simulink model "Linearisation_AleixGranero_MichalSzabo"  (R2021b)
settings: Solver=ode3  StartTime=0.0  StopTime=1000  FixedStep=Ts  RelTol=1e-3  EnableMultiTasking=on
values from neighbouring files (symbols this model uses):
  A = [K1   0 -K3   0 ... (first row only)    [Discretisation_MichalSzabo_AleixGranero.m]    (also in Linearisation_MichalSzabo_AleixGranero.m)
  A1 = 28    [Discretisation_MichalSzabo_AleixGranero.m]    (also in Linearisation_MichalSzabo_AleixGranero.m)
  a1 = 0.071    [Discretisation_MichalSzabo_AleixGranero.m]    (also in Linearisation_MichalSzabo_AleixGranero.m)
  A2 = 28    [Discretisation_MichalSzabo_AleixGranero.m]    (also in Linearisation_MichalSzabo_AleixGranero.m)
  a2 = 0.071    [Discretisation_MichalSzabo_AleixGranero.m]    (also in Linearisation_MichalSzabo_AleixGranero.m)
  a3 = 0.071    [Discretisation_MichalSzabo_AleixGranero.m]    (also in Linearisation_MichalSzabo_AleixGranero.m)
  A3 = 28    [Discretisation_MichalSzabo_AleixGranero.m]    (also in Linearisation_MichalSzabo_AleixGranero.m)
  a4 = 0.071    [Discretisation_MichalSzabo_AleixGranero.m]    (also in Linearisation_MichalSzabo_AleixGranero.m)
  A4 = 28    [Discretisation_MichalSzabo_AleixGranero.m]    (also in Linearisation_MichalSzabo_AleixGranero.m)
  B = [J2 0 ... (first row only)    [Discretisation_MichalSzabo_AleixGranero.m]    (also in Linearisation_MichalSzabo_AleixGranero.m)
  C = eye(4)    [Discretisation_MichalSzabo_AleixGranero.m]    (also in Linearisation_MichalSzabo_AleixGranero.m)
  D = zeros(4,2)    [Discretisation_MichalSzabo_AleixGranero.m]    (also in Linearisation_MichalSzabo_AleixGranero.m)
  g = 981    [Discretisation_MichalSzabo_AleixGranero.m]    (also in Linearisation_MichalSzabo_AleixGranero.m)
  gamma1 = 0.7    [Discretisation_MichalSzabo_AleixGranero.m]    (also in Linearisation_MichalSzabo_AleixGranero.m)
  gamma2 = 0.7    [Discretisation_MichalSzabo_AleixGranero.m]    (also in Linearisation_MichalSzabo_AleixGranero.m)
  h10 = 1/(2*g)*(a3/a1 * sqrt(2*g*h30)+gamma1*k1/a1*v10)^2    [Discretisation_MichalSzabo_AleixGranero.m]    (also in Linearisation_MichalSzabo_AleixGranero.m)
  h20 = 1/(2*g)*(a4/a2 * sqrt(2*g*h40)+gamma2*k1/a2*v20)^2    [Discretisation_MichalSzabo_AleixGranero.m]    (also in Linearisation_MichalSzabo_AleixGranero.m)
  h30 = 1/(2*g)*((1-gamma2)*k2*v20/a3)^2    (= 0.40362240636)    [Discretisation_MichalSzabo_AleixGranero.m]    (also in Linearisation_MichalSzabo_AleixGranero.m)
  h40 = 1/(2*g)*((1-gamma1)*k2*v10/a4)^2    (= 0.40362240636)    [Discretisation_MichalSzabo_AleixGranero.m]    (also in Linearisation_MichalSzabo_AleixGranero.m)
  k1 = 3.33    [Discretisation_MichalSzabo_AleixGranero.m]    (also in Linearisation_MichalSzabo_AleixGranero.m)
  k2 = 3.33    [Discretisation_MichalSzabo_AleixGranero.m]    (also in Linearisation_MichalSzabo_AleixGranero.m)
  t1 = 200    [Discretisation_MichalSzabo_AleixGranero.m]    (also in Linearisation_MichalSzabo_AleixGranero.m)
  t2 = 400    [Discretisation_MichalSzabo_AleixGranero.m]    (also in Linearisation_MichalSzabo_AleixGranero.m)
  v10 = 2    [Discretisation_MichalSzabo_AleixGranero.m]    (also in Linearisation_MichalSzabo_AleixGranero.m)
  v11 = 2.2    [Discretisation_MichalSzabo_AleixGranero.m]    (also in Linearisation_MichalSzabo_AleixGranero.m)
  v20 = 2    [Discretisation_MichalSzabo_AleixGranero.m]    (also in Linearisation_MichalSzabo_AleixGranero.m)
  v22 = 1.8    [Discretisation_MichalSzabo_AleixGranero.m]    (also in Linearisation_MichalSzabo_AleixGranero.m)
settings Model: Creator=as  LastModifiedBy=szmis
settings SolverCC: AlgebraicLoopSolver=TrustRegion
settings DataIOCC: LimitDataPoints=on  SaveFormat=Array  SignalLoggingSaveFormat=ModelDataLogs  ReturnWorkspaceOutputs=off
settings OptimizationCC: LifeSpan=inf
settings DebuggingCC: SaveWithParameterizedLinksMsg=none  UnderspecifiedInitializationDetection=Classic  MergeDetectMultiDrivingBlocksExec=none  SolverPrmCheckMsg=warning  FcnCallInpInsideContextMsg=warning  SFUnexpectedBacktrackingDiag=warning  SFNoUnconditionalDefaultTransitionDiag=warning  SFExecutionAtInitializationDiag=none  SFMachineParentedDataDiag=warning  ArithmeticOperatorsInVariantConditions=warning
settings HardwareCC: ProdBitPerPointer=32  ProdBitPerSizeT=32  ProdBitPerPtrDiffT=32  ProdLargestAtomicFloat=None  ProdIntDivRoundTo=Undefined  ProdEndianess=Unspecified  ProdWordSize=32  ProdHWDeviceType=32-bit Generic
settings ModelReferenceCC: PropagateSignalLabelsOutOfModel=off
settings SFSimCC: SimUseLocalCustomCode=off  CustomCodeUndefinedFunction=UseInterfaceOnly
settings RTWCC: RTWUseLocalCustomCode=off
settings CodeAppCC: StateflowObjectComments=on
settings GRTTargetCC: TargetLangStandard=C89/C90 (ANSI)  CombineOutputUpdateFcns=off  GRTInterface=on
settings ConfigComp: CovMetricSettings=dw  CovSaveCumulativeToWorkspaceVar=on  CovSaveSingleToWorkspaceVar=on  CovExternalEMLEnable=off

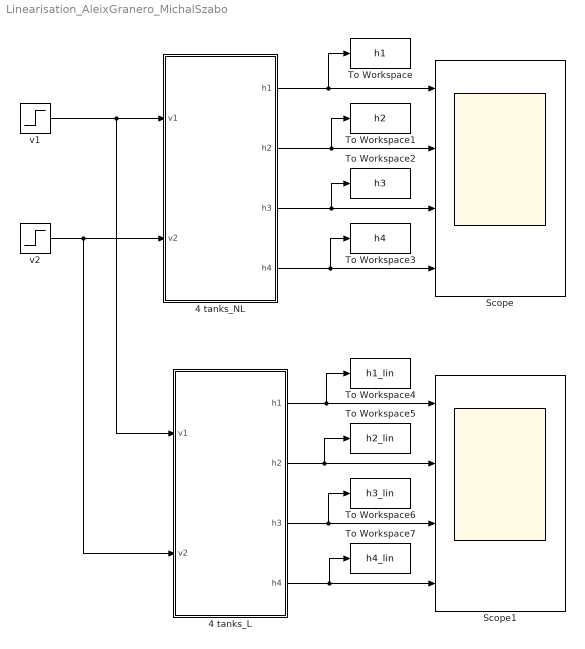
== system Linearisation_AleixGranero_MichalSzabo ==
  4 tanks_L : Subsystem
  4 tanks_NL : Subsystem
  Scope : Scope  NumInputPorts=4
  Scope1 : Scope  NumInputPorts=4
  To Workspace : ToWorkspace  VariableName=h1  SampleTime=-1
  To Workspace1 : ToWorkspace  VariableName=h2  SampleTime=-1
  To Workspace2 : ToWorkspace  VariableName=h3  SampleTime=-1
  To Workspace3 : ToWorkspace  VariableName=h4  SampleTime=-1
  To Workspace4 : ToWorkspace  VariableName=h1_lin  SampleTime=-1
  To Workspace5 : ToWorkspace  VariableName=h2_lin  SampleTime=-1
  To Workspace6 : ToWorkspace  VariableName=h3_lin  SampleTime=-1
  To Workspace7 : ToWorkspace  VariableName=h4_lin  SampleTime=-1
  v1 : Step  Time=t1  Before=v10  After=v11  SampleTime=0
  v2 : Step  Time=t2  Before=v20  After=v22  SampleTime=0
  wires:
  4 tanks_L/4("h4 ") -> To Workspace7/1, Scope1/4
  4 tanks_NL/4("h4 ") -> To Workspace3/1, Scope/4
  4 tanks_L/2("h2 ") -> To Workspace5/1, Scope1/2
  4 tanks_NL/1("h1 ") -> To Workspace/1, Scope/1
  4 tanks_L/1("h1 ") -> To Workspace4/1, Scope1/1
  4 tanks_L/3("h3 ") -> To Workspace6/1, Scope1/3
  v2/1 -> 4 tanks_L/2(v2), 4 tanks_NL/2(v2)
  v1/1 -> 4 tanks_L/1(v1), 4 tanks_NL/1(v1)
  4 tanks_NL/3("h3 ") -> To Workspace2/1, Scope/3
  4 tanks_NL/2("h2 ") -> To Workspace1/1, Scope/2

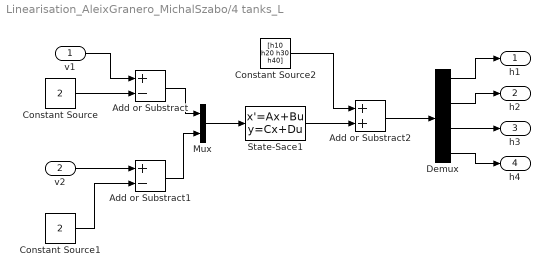
== system Linearisation_AleixGranero_MichalSzabo/4 tanks_L ==
  v1 : Inport
  v2 : Inport  Port=2
  Add or Substract : Sum  Inputs=+-
  Add or Substract1 : Sum  Inputs=+-
  Add or Substract2 : Sum
  Constant Source : Constant  Value=2
  Constant Source1 : Constant  Value=2
  Constant Source2 : Constant  Value=[h10 h20 h30 h40]
  Demux : Demux
  Mux : Mux  Inputs=2
  State-Sace1 : StateSpace  A=A  B=B  C=C  D=D  InitialCondition=0
  "h1 " : Outport
  "h2 " : Outport  Port=2
  "h3 " : Outport  Port=3
  "h4 " : Outport  Port=4
  wires:
  Mux/1 -> State-Sace1/1
  Constant Source/1 -> Add or Substract/2
  v1/1 -> Add or Substract/1
  v2/1 -> Add or Substract1/1
  Constant Source1/1 -> Add or Substract1/2
  Add or Substract/1 -> Mux/1
  Add or Substract1/1 -> Mux/2
  State-Sace1/1 -> Add or Substract2/2
  Add or Substract2/1 -> Demux/1
  Demux/1 -> "h1 "/1
  Demux/2 -> "h2 "/1
  Demux/3 -> "h3 "/1
  Demux/4 -> "h4 "/1
  Constant Source2/1 -> Add or Substract2/1

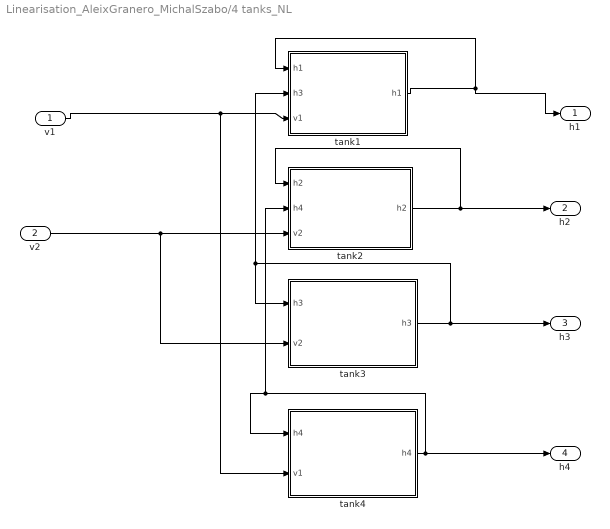
== system Linearisation_AleixGranero_MichalSzabo/4 tanks_NL ==
  v1 : Inport
  v2 : Inport  Port=2
  tank1 : Subsystem
  tank2 : Subsystem
  tank3 : Subsystem
  tank4 : Subsystem
  "h1 " : Outport
  "h2 " : Outport  Port=2
  "h3 " : Outport  Port=3
  "h4 " : Outport  Port=4
  wires:
  tank4/1("h4 ") -> tank4/1(h4), tank2/2(h4), "h4 "/1
  tank3/1("h3 ") -> tank3/1(h3), tank1/2(h3), "h3 "/1
  v2/1 -> tank2/3(v2), tank3/2(v2)
  tank2/1("h2 ") -> tank2/1(h2), "h2 "/1
  v1/1 -> tank1/3(v1), tank4/2(v1)
  tank1/1("h1 ") -> "h1 "/1, tank1/1(h1)

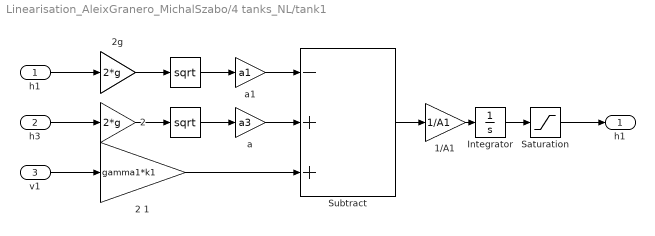
== system Linearisation_AleixGranero_MichalSzabo/4 tanks_NL/tank1 ==
  h1 : Inport
  h3 : Inport  Port=2
  v1 : Inport  Port=3
  " " : Math  Operator=sqrt  SignedPower=on  SaturateOnIntegerOverflow=on
  "   " : Math  Operator=sqrt  SignedPower=on  SaturateOnIntegerOverflow=on
  1/A1 : Gain  Gain=1/A1
  "2 " : Gain  Gain=2*g
  2 1 : Gain  Gain=gamma1*k1
  2g : Gain  Gain=2*g
  Integrator : Integrator  InitialCondition=h10
  Saturation : Saturate  UpperLimit=15  LowerLimit=0
  Subtract : Sum  Inputs=-++
  a : Gain  Gain=a3
  a1 : Gain  Gain=a1
  "h1 " : Outport
  wires:
  " "/1 -> a1/1
  2g/1 -> " "/1
  a1/1 -> Subtract/1
  h1/1 -> 2g/1
  "   "/1 -> a/1
  "2 "/1 -> "   "/1
  a/1 -> Subtract/2
  h3/1 -> "2 "/1
  2 1/1 -> Subtract/3
  v1/1 -> 2 1/1
  1/A1/1 -> Integrator/1
  Saturation/1 -> "h1 "/1
  Integrator/1 -> Saturation/1
  Subtract/1 -> 1/A1/1

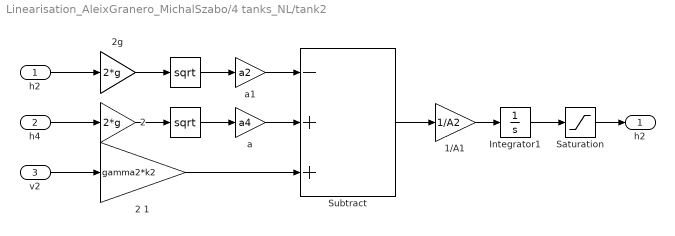
== system Linearisation_AleixGranero_MichalSzabo/4 tanks_NL/tank2 ==
  h2 : Inport
  h4 : Inport  Port=2
  v2 : Inport  Port=3
  " " : Math  Operator=sqrt  SignedPower=on  SaturateOnIntegerOverflow=on
  "   " : Math  Operator=sqrt  SignedPower=on  SaturateOnIntegerOverflow=on
  1/A1 : Gain  Gain=1/A2
  "2 " : Gain  Gain=2*g
  2 1 : Gain  Gain=gamma2*k2
  2g : Gain  Gain=2*g
  Integrator1 : Integrator  InitialCondition=h20
  Saturation : Saturate  UpperLimit=15  LowerLimit=0
  Subtract : Sum  Inputs=-++
  a : Gain  Gain=a4
  a1 : Gain  Gain=a2
  "h2 " : Outport
  wires:
  1/A1/1 -> Integrator1/1
  v2/1 -> 2 1/1
  2 1/1 -> Subtract/3
  h4/1 -> "2 "/1
  a/1 -> Subtract/2
  "2 "/1 -> "   "/1
  "   "/1 -> a/1
  h2/1 -> 2g/1
  a1/1 -> Subtract/1
  2g/1 -> " "/1
  " "/1 -> a1/1
  Saturation/1 -> "h2 "/1
  Integrator1/1 -> Saturation/1
  Subtract/1 -> 1/A1/1

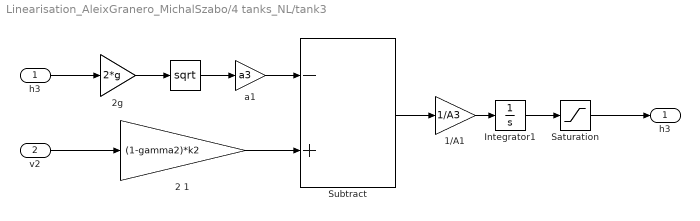
== system Linearisation_AleixGranero_MichalSzabo/4 tanks_NL/tank3 ==
  h3 : Inport
  v2 : Inport  Port=2
  " " : Math  Operator=sqrt  SignedPower=on  SaturateOnIntegerOverflow=on
  1/A1 : Gain  Gain=1/A3
  2 1 : Gain  Gain=(1-gamma2)*k2
  2g : Gain  Gain=2*g
  Integrator1 : Integrator  InitialCondition=h30
  Saturation : Saturate  UpperLimit=15  LowerLimit=0
  Subtract : Sum  Inputs=-+
  a1 : Gain  Gain=a3
  "h3 " : Outport
  wires:
  " "/1 -> a1/1
  2g/1 -> " "/1
  a1/1 -> Subtract/1
  h3/1 -> 2g/1
  2 1/1 -> Subtract/2
  v2/1 -> 2 1/1
  1/A1/1 -> Integrator1/1
  Saturation/1 -> "h3 "/1
  Subtract/1 -> 1/A1/1
  Integrator1/1 -> Saturation/1

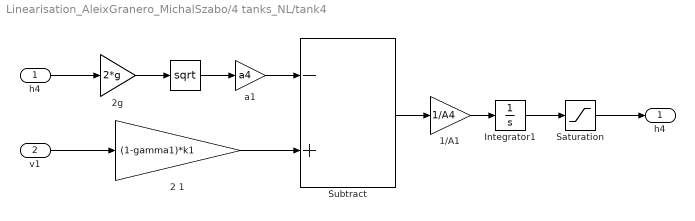
== system Linearisation_AleixGranero_MichalSzabo/4 tanks_NL/tank4 ==
  h4 : Inport
  v1 : Inport  Port=2
  " " : Math  Operator=sqrt  SignedPower=on  SaturateOnIntegerOverflow=on
  1/A1 : Gain  Gain=1/A4
  2 1 : Gain  Gain=(1-gamma1)*k1
  2g : Gain  Gain=2*g
  Integrator1 : Integrator  InitialCondition=h40
  Saturation : Saturate  UpperLimit=15  LowerLimit=0
  Subtract : Sum  Inputs=-+
  a1 : Gain  Gain=a4
  "h4 " : Outport
  wires:
  1/A1/1 -> Integrator1/1
  v1/1 -> 2 1/1
  2 1/1 -> Subtract/2
  h4/1 -> 2g/1
  a1/1 -> Subtract/1
  2g/1 -> " "/1
  " "/1 -> a1/1
  Saturation/1 -> "h4 "/1
  Subtract/1 -> 1/A1/1
  Integrator1/1 -> Saturation/1
